simulink model "EXTENDEDKALMANFINAL2021abid"  (R2021a)
settings: Solver=ode4  StartTime=0.0  StopTime=200  FixedStep=0.02  RelTol=1e-3
libraries: commchan3 x2
(part 3 of 4)

== matlab function EXTENDEDKALMANFINAL2021abid/MATLAB Function2 ==
  data: xhatp input; Pp input; y input; u input; xhat output; P output
function [xhat, P]= fcn(xhatp, Pp, y, u)
x4=xhatp(4);
x5=xhatp(5);
x1=xhatp(1);
x2=xhatp(2);
x3=xhatp(3);

A=[                                                                                                                                                                                                                                                                                                                                                                             (x5/x4 + 5)/(1500000*x4) - 67/(505000*x4) + 1,                                                                                                                                                                                                                                                                                                                                                                                                                                                                                                                             ((x5/x4 + 5)*(x5/(20*x4) + 1/x4))/1500000 - x5/(150000*x4) - 1/(7500*x4) + 1/50,                                                                                                                                                                                                                                                                                                                                                                                                                                                                                                                                                  ((x5/x4 + 5)*(x5/(100*x4) - 19/20))/1500000 - (7*x5)/(10000000*x4) - 1/(1515000*x4) + 59/300000,                                                                                                                                                                                                                                                                                                                                                                                                                                                                                                                                                                                                                                                                                                                                                                                                                                                                                                                                                                                                                                                                                                                                                                                                                                                                                                                                                                                                                                                                                                                                                                                                                                                                                                                                                                                                                                                                                                                                                                                                                                                                                                                                                                                                                                                                                                                                                                                                                                                                                                                                                                                                                                                                                                                                                                                                                                                                                                                                                                                                                                                                                                                                                                                                                                       (x2*((5*x5)/x4^2 + 100/x4^2))/1500000 + (((5*x5)/x4^2 + 10000/(101*x4^2))*(x2 + x3/100))/1500000 - ((x5/x4 + 5)*((x2*((5*x5)/x4^2 + 100/x4^2))/100 + u/(20*x4^2) + x1/x4^2 + (x3*x5)/(100*x4^2)))/1500000 + (67*u)/(10100000*x4^2) + x1/(15000*x4^2) + (x1 + x2/100)/(15150*x4^2) + (x3*x5)/(1500000*x4^2) - (x5*((x2*((5*x5)/x4 + 100/x4))/100 - x3 + u/(20*x4) + x1/x4 + (x3*(x5/x4 + 5))/100))/(1500000*x4^2),                                                                                                                                                                                                                                                                                                                                                                                                                                                                                                                                                                                                                                                                                                                                                                                                                                                                                                                                                                                                                                                                                                                                                                                                                                                                                                                                                                                                                                                                                                                                                                                                                                                                                                                                                                                                                                                                                                                                                                                                                                                                                                                                                                            ((x5/x4 + 5)*(x2/(20*x4) + x3/(100*x4)))/1500000 - x2/(300000*x4) - x3/(1500000*x4) + ((x2*((5*x5)/x4 + 100/x4))/100 - x3 + u/(20*x4) + x1/x4 + (x3*(x5/x4 + 5))/100)/(1500000*x4) - (x2 + x3/100)/(300000*x4);
                                                                                                                                                                                                                                                               (x5/x4 + 5)/(15000*x4) - ((x5/x4 + 5)*((x5/x4 + 5)/(100*x4) - 100/(101*x4)))/15000 + ((5*x5)/x4 + 1000000/(10101*x4))/(1500000*x4) - 3040301/(153030150*x4),                                                                                                                                                                                                                                                                                                                                                                 ((x5/x4 + 5)*(x5/(20*x4) + 1/x4))/15000 + ((x5/x4 + 5)*(x5/(20*x4) - ((x5/x4 + 5)*(x5/(20*x4) + 1/x4))/100 + 1/x4))/15000 - x5/(1500*x4) - 10151/(757575*x4) + (((5*x5)/x4 + 1000000/(10101*x4))*(x5/(2000*x4) + 1/(100*x4) - 1))/15000 + 1,                                                                                                                                                                                                                                                                                                                                                                               ((x5/x4 + 5)*(x5/(100*x4) - 19/20))/15000 - ((x5/x4 + 5)*(((x5/x4 + 5)*(x5/(100*x4) - 19/20))/100 - x5/(2000*x4) - 1/(101*x4) + 1))/15000 - (7*x5)/(100000*x4) + ((x5/(10000*x4) - 19/2000)*((5*x5)/x4 + 1000000/(10101*x4)))/15000 - 5101/(76515075*x4) + 59/3000,                                                                                                                                                                                                                                                                                                                                                                                                                                                                                                                                                                                                                                                                                                                                                                                                                                                                                                                                                                                                                                                                                                                                                                                                                                                                                                                                                                                                                                                                                                                                                                                                                                                                                                                                                                                                                                                                                                                                                                                                                                                                                                                                                                                                                                                                                                                        (x2*((5*x5)/x4^2 + 100/x4^2))/15000 - (((5*x5)/x4^2 + 1000000/(10101*x4^2))*((x2*((5*x5)/x4 + 100/x4))/10000 - x3/100 - x2 + u/(2000*x4) + x1/(100*x4) + (x3*(x5/x4 + 5))/10000))/15000 + (((5*x5)/x4^2 + 10000/(101*x4^2))*(x2 + x3/100))/15000 - ((x5/x4 + 5)*((((5*x5)/x4^2 + 10000/(101*x4^2))*(x2 + x3/100))/100 - ((x5/x4 + 5)*((x2*((5*x5)/x4^2 + 100/x4^2))/100 + u/(20*x4^2) + x1/x4^2 + (x3*x5)/(100*x4^2)))/100 + (5*u)/(101*x4^2) + (100*(x1 + x2/100))/(101*x4^2) - (x5*((x2*((5*x5)/x4 + 100/x4))/100 - x3 + u/(20*x4) + x1/x4 + (x3*(x5/x4 + 5))/100))/(100*x4^2)))/15000 - ((x5/x4 + 5)*((x2*((5*x5)/x4^2 + 100/x4^2))/100 + u/(20*x4^2) + x1/x4^2 + (x3*x5)/(100*x4^2)))/15000 - (((5*x5)/x4 + 1000000/(10101*x4))*((x2*((5*x5)/x4^2 + 100/x4^2))/10000 + u/(2000*x4^2) + x1/(100*x4^2) + (x3*x5)/(10000*x4^2)))/15000 + (3040301*u)/(3060603000*x4^2) + x1/(150*x4^2) + (200*(x1 + x2/100 + x3/10000))/(30303*x4^2) + (2*(x1 + x2/100))/(303*x4^2) + (x3*x5)/(15000*x4^2) - (x5*((x2*((5*x5)/x4 + 100/x4))/100 - x3 + u/(20*x4) + x1/x4 + (x3*(x5/x4 + 5))/100))/(15000*x4^2) - (x5*((((5*x5)/x4 + 10000/(101*x4))*(x2 + x3/100))/100 - ((x5/x4 + 5)*((x2*((5*x5)/x4 + 100/x4))/100 - x3 + u/(20*x4) + x1/x4 + (x3*(x5/x4 + 5))/100))/100 - x3 + (5*u)/(101*x4) + (100*(x1 + x2/100))/(101*x4)))/(15000*x4^2),                                                                                                                                                                                                                                                                                                                                                                                                                                                                                                                                                                                                                                                                                                                                                                                                                                                                                                                                                                                                                                                                                                                                                                                                                                                                                                                                                                                                                                                                                                                                                                          ((x5/x4 + 5)*(x2/(20*x4) + x3/(100*x4)))/15000 + ((((5*x5)/x4 + 10000/(101*x4))*(x2 + x3/100))/100 - ((x5/x4 + 5)*((x2*((5*x5)/x4 + 100/x4))/100 - x3 + u/(20*x4) + x1/x4 + (x3*(x5/x4 + 5))/100))/100 - x3 + (5*u)/(101*x4) + (100*(x1 + x2/100))/(101*x4))/(15000*x4) + (((5*x5)/x4 + 1000000/(10101*x4))*(x2/(2000*x4) + x3/(10000*x4)))/15000 + ((x2*((5*x5)/x4 + 100/x4))/10000 - x3/100 - x2 + u/(2000*x4) + x1/(100*x4) + (x3*(x5/x4 + 5))/10000)/(3000*x4) - ((x5/x4 + 5)*(((x5/x4 + 5)*(x2/(20*x4) + x3/(100*x4)))/100 + ((x2*((5*x5)/x4 + 100/x4))/100 - x3 + u/(20*x4) + x1/x4 + (x3*(x5/x4 + 5))/100)/(100*x4) - (x2 + x3/100)/(20*x4)))/15000 - x2/(3000*x4) - x3/(15000*x4) + ((x2*((5*x5)/x4 + 100/x4))/100 - x3 + u/(20*x4) + x1/x4 + (x3*(x5/x4 + 5))/100)/(15000*x4) - (x2 + x3/100)/(3000*x4);
(x5/x4 + 5)/(150*x4) - ((x5/x4 + 5)*((x5/x4 + 5)/(100*x4) - 100/(101*x4)))/150 + ((5*x5)/x4 + 1000000/(10101*x4))/(15000*x4) - (((5*x5)/x4 + 50000000/(510101*x4))*((x5/x4 + 5)/(5000*x4) - 2/(101*x4)))/300 + ((x5/x4 + 5)*(((x5/x4 + 5)*((x5/x4 + 5)/(100*x4) - 100/(101*x4)))/50 - ((5*x5)/x4 + 1000000/(10101*x4))/(5000*x4) + 20000/(10101*x4)))/300 + (500000*(1/(5000*x4) - 1))/(1530303*x4) - 5060401/(3060603*x4), ((x5/x4 + 5)*(x5/(20*x4) + 1/x4))/150 - (((5*x5)/x4 + 50000000/(510101*x4))*(((x5/x4 + 5)*(x5/(20*x4) + 1/x4))/5000 - x5/(1000*x4) - 1/(50*x4) + 1))/300 + (500000*(x5/(100000*x4) + 1/(5000*x4) - 1/50))/(1530303*x4) - ((x5/x4 + 5)*(((x5/x4 + 5)*(x5/(20*x4) - ((x5/x4 + 5)*(x5/(20*x4) + 1/x4))/100 + 1/x4))/50 - 200/(10101*x4) + (((5*x5)/x4 + 1000000/(10101*x4))*(x5/(2000*x4) + 1/(100*x4) - 1))/50))/300 + ((x5/x4 + 5)*(x5/(20*x4) - ((x5/x4 + 5)*(x5/(20*x4) + 1/x4))/100 + 1/x4))/150 - x5/(20*x4) - 30503/(30303*x4) + (((5*x5)/x4 + 1000000/(10101*x4))*(x5/(2000*x4) + 1/(100*x4) - 1))/150, (500000*(x5/(500000*x4) - 19/100000))/(1530303*x4) - ((x5/x4 + 5)*(((x5/x4 + 5)*(x5/(100*x4) - 19/20))/100 - x5/(2000*x4) - 1/(101*x4) + 1))/150 - (((5*x5)/x4 + 50000000/(510101*x4))*(((x5/x4 + 5)*(x5/(100*x4) - 19/20))/5000 - x5/(100000*x4) - 1/(5050*x4) + 1/50))/300 + ((x5/x4 + 5)*(x5/(100*x4) - 19/20))/150 - (11*x5)/(3000*x4) + ((x5/(10000*x4) - 19/2000)*((5*x5)/x4 + 1000000/(10101*x4)))/150 - 20404/(3060603*x4) + ((x5/x4 + 5)*(((x5/x4 + 5)*(((x5/x4 + 5)*(x5/(100*x4) - 19/20))/100 - x5/(2000*x4) - 1/(101*x4) + 1))/50 - ((x5/(10000*x4) - 19/2000)*((5*x5)/x4 + 1000000/(10101*x4)))/50 + 2/(10101*x4) - 1))/300 + 59/60, ((x5/x4 + 5)*((((5*x5)/x4^2 + 1000000/(10101*x4^2))*((x2*((5*x5)/x4 + 100/x4))/10000 - x3/100 - x2 + u/(2000*x4) + x1/(100*x4) + (x3*(x5/x4 + 5))/10000))/50 + ((x5/x4 + 5)*((((5*x5)/x4^2 + 10000/(101*x4^2))*(x2 + x3/100))/100 - ((x5/x4 + 5)*((x2*((5*x5)/x4^2 + 100/x4^2))/100 + u/(20*x4^2) + x1/x4^2 + (x3*x5)/(100*x4^2)))/100 + (5*u)/(101*x4^2) + (100*(x1 + x2/100))/(101*x4^2) - (x5*((x2*((5*x5)/x4 + 100/x4))/100 - x3 + u/(20*x4) + x1/x4 + (x3*(x5/x4 + 5))/100))/(100*x4^2)))/50 + (((5*x5)/x4 + 1000000/(10101*x4))*((x2*((5*x5)/x4^2 + 100/x4^2))/10000 + u/(2000*x4^2) + x1/(100*x4^2) + (x3*x5)/(10000*x4^2)))/50 - (1000*u)/(10101*x4^2) - (20000*(x1 + x2/100 + x3/10000))/(10101*x4^2) + (x5*((((5*x5)/x4 + 10000/(101*x4))*(x2 + x3/100))/100 - ((x5/x4 + 5)*((x2*((5*x5)/x4 + 100/x4))/100 - x3 + u/(20*x4) + x1/x4 + (x3*(x5/x4 + 5))/100))/100 - x3 + (5*u)/(101*x4) + (100*(x1 + x2/100))/(101*x4)))/(50*x4^2)))/300 - (((5*x5)/x4^2 + 1000000/(10101*x4^2))*((x2*((5*x5)/x4 + 100/x4))/10000 - x3/100 - x2 + u/(2000*x4) + x1/(100*x4) + (x3*(x5/x4 + 5))/10000))/150 + (x2*((5*x5)/x4^2 + 100/x4^2))/300 - (500000*((x2*((5*x5)/x4^2 + 100/x4^2))/500000 + u/(100000*x4^2) + x1/(5000*x4^2) + (x3*x5)/(500000*x4^2)))/(1530303*x4) + (((5*x5)/x4^2 + 50000000/(510101*x4^2))*(x2 + x3/50 + ((x5/x4 + 5)*((x2*((5*x5)/x4 + 100/x4))/100 - x3 + u/(20*x4) + x1/x4 + (x3*(x5/x4 + 5))/100))/5000 - (((5*x5)/x4 + 10000/(101*x4))*(x2 + x3/100))/5000 - u/(1010*x4) - (2*(x1 + x2/100))/(101*x4)))/300 + (((5*x5)/x4^2 + 10000/(101*x4^2))*(x2 + x3/100))/150 - ((x5/x4 + 5)*((((5*x5)/x4^2 + 10000/(101*x4^2))*(x2 + x3/100))/100 - ((x5/x4 + 5)*((x2*((5*x5)/x4^2 + 100/x4^2))/100 + u/(20*x4^2) + x1/x4^2 + (x3*x5)/(100*x4^2)))/100 + (5*u)/(101*x4^2) + (100*(x1 + x2/100))/(101*x4^2) - (x5*((x2*((5*x5)/x4 + 100/x4))/100 - x3 + u/(20*x4) + x1/x4 + (x3*(x5/x4 + 5))/100))/(100*x4^2)))/150 - ((x5/x4 + 5)*((x2*((5*x5)/x4^2 + 100/x4^2))/100 + u/(20*x4^2) + x1/x4^2 + (x3*x5)/(100*x4^2)))/150 - (500000*((x2*((5*x5)/x4 + 100/x4))/500000 - x2/50 - x3/5000 - x1 + u/(100000*x4) + x1/(5000*x4) + (x3*(x5/x4 + 5))/500000))/(1530303*x4^2) - (((5*x5)/x4 + 50000000/(510101*x4))*((((5*x5)/x4^2 + 10000/(101*x4^2))*(x2 + x3/100))/5000 - ((x5/x4 + 5)*((x2*((5*x5)/x4^2 + 100/x4^2))/100 + u/(20*x4^2) + x1/x4^2 + (x3*x5)/(100*x4^2)))/5000 + u/(1010*x4^2) + (2*(x1 + x2/100))/(101*x4^2) - (x5*((x2*((5*x5)/x4 + 100/x4))/100 - x3 + u/(20*x4) + x1/x4 + (x3*(x5/x4 + 5))/100))/(5000*x4^2)))/300 - (((5*x5)/x4 + 1000000/(10101*x4))*((x2*((5*x5)/x4^2 + 100/x4^2))/10000 + u/(2000*x4^2) + x1/(100*x4^2) + (x3*x5)/(10000*x4^2)))/150 + (3091416110501*u)/(31224333018060*x4^2) + x1/(3*x4^2) + (20000*(x1 + x2/100 + x3/10000))/(30303*x4^2) + (200*(x1 + x2/100))/(303*x4^2) + (x3*x5)/(300*x4^2) - (x5*((x2*((5*x5)/x4 + 100/x4))/100 - x3 + u/(20*x4) + x1/x4 + (x3*(x5/x4 + 5))/100))/(150*x4^2) + (x5*(x3 + (((5*x5)/x4 + 1000000/(10101*x4))*((x2*((5*x5)/x4 + 100/x4))/10000 - x3/100 - x2 + u/(2000*x4) + x1/(100*x4) + (x3*(x5/x4 + 5))/10000))/50 + ((x5/x4 + 5)*((((5*x5)/x4 + 10000/(101*x4))*(x2 + x3/100))/100 - ((x5/x4 + 5)*((x2*((5*x5)/x4 + 100/x4))/100 - x3 + u/(20*x4) + x1/x4 + (x3*(x5/x4 + 5))/100))/100 - x3 + (5*u)/(101*x4) + (100*(x1 + x2/100))/(101*x4)))/50 - (1000*u)/(10101*x4) - (20000*(x1 + x2/100 + x3/10000))/(10101*x4)))/(300*x4^2) - (x5*((((5*x5)/x4 + 10000/(101*x4))*(x2 + x3/100))/100 - ((x5/x4 + 5)*((x2*((5*x5)/x4 + 100/x4))/100 - x3 + u/(20*x4) + x1/x4 + (x3*(x5/x4 + 5))/100))/100 - x3 + (5*u)/(101*x4) + (100*(x1 + x2/100))/(101*x4)))/(150*x4^2), ((x5/x4 + 5)*(x2/(20*x4) + x3/(100*x4)))/150 - (x3 + (((5*x5)/x4 + 1000000/(10101*x4))*((x2*((5*x5)/x4 + 100/x4))/10000 - x3/100 - x2 + u/(2000*x4) + x1/(100*x4) + (x3*(x5/x4 + 5))/10000))/50 + ((x5/x4 + 5)*((((5*x5)/x4 + 10000/(101*x4))*(x2 + x3/100))/100 - ((x5/x4 + 5)*((x2*((5*x5)/x4 + 100/x4))/100 - x3 + u/(20*x4) + x1/x4 + (x3*(x5/x4 + 5))/100))/100 - x3 + (5*u)/(101*x4) + (100*(x1 + x2/100))/(101*x4)))/50 - (1000*u)/(10101*x4) - (20000*(x1 + x2/100 + x3/10000))/(10101*x4))/(300*x4) + ((((5*x5)/x4 + 10000/(101*x4))*(x2 + x3/100))/100 - ((x5/x4 + 5)*((x2*((5*x5)/x4 + 100/x4))/100 - x3 + u/(20*x4) + x1/x4 + (x3*(x5/x4 + 5))/100))/100 - x3 + (5*u)/(101*x4) + (100*(x1 + x2/100))/(101*x4))/(150*x4) + (((5*x5)/x4 + 1000000/(10101*x4))*(x2/(2000*x4) + x3/(10000*x4)))/150 + ((x2*((5*x5)/x4 + 100/x4))/10000 - x3/100 - x2 + u/(2000*x4) + x1/(100*x4) + (x3*(x5/x4 + 5))/10000)/(30*x4) - ((x5/x4 + 5)*(((x5/x4 + 5)*(x2/(20*x4) + x3/(100*x4)))/100 + ((x2*((5*x5)/x4 + 100/x4))/100 - x3 + u/(20*x4) + x1/x4 + (x3*(x5/x4 + 5))/100)/(100*x4) - (x2 + x3/100)/(20*x4)))/150 - x2/(60*x4) - x3/(300*x4) + ((x2*((5*x5)/x4 + 100/x4))/100 - x3 + u/(20*x4) + x1/x4 + (x3*(x5/x4 + 5))/100)/(150*x4) - (x2 + x3/50 + ((x5/x4 + 5)*((x2*((5*x5)/x4 + 100/x4))/100 - x3 + u/(20*x4) + x1/x4 + (x3*(x5/x4 + 5))/100))/5000 - (((5*x5)/x4 + 10000/(101*x4))*(x2 + x3/100))/5000 - u/(1010*x4) - (2*(x1 + x2/100))/(101*x4))/(60*x4) - ((x5/x4 + 5)*(((((5*x5)/x4 + 10000/(101*x4))*(x2 + x3/100))/100 - ((x5/x4 + 5)*((x2*((5*x5)/x4 + 100/x4))/100 - x3 + u/(20*x4) + x1/x4 + (x3*(x5/x4 + 5))/100))/100 - x3 + (5*u)/(101*x4) + (100*(x1 + x2/100))/(101*x4))/(50*x4) + (((5*x5)/x4 + 1000000/(10101*x4))*(x2/(2000*x4) + x3/(10000*x4)))/50 + ((x2*((5*x5)/x4 + 100/x4))/10000 - x3/100 - x2 + u/(2000*x4) + x1/(100*x4) + (x3*(x5/x4 + 5))/10000)/(10*x4) - ((x5/x4 + 5)*(((x5/x4 + 5)*(x2/(20*x4) + x3/(100*x4)))/100 + ((x2*((5*x5)/x4 + 100/x4))/100 - x3 + u/(20*x4) + x1/x4 + (x3*(x5/x4 + 5))/100)/(100*x4) - (x2 + x3/100)/(20*x4)))/50))/300 - (((5*x5)/x4 + 50000000/(510101*x4))*(((x5/x4 + 5)*(x2/(20*x4) + x3/(100*x4)))/5000 + ((x2*((5*x5)/x4 + 100/x4))/100 - x3 + u/(20*x4) + x1/x4 + (x3*(x5/x4 + 5))/100)/(5000*x4) - (x2 + x3/100)/(1000*x4)))/300 - (x2 + x3/100)/(30*x4) + (500000*(x2/(100000*x4) + x3/(500000*x4)))/(1530303*x4);
                                                                                                                                                                                                                                                                                                                                                                                                                         0,                                                                                                                                                                                                                                                                                                                                                                                                                                                                                                                                                                                                           0,                                                                                                                                                                                                                                                                                                                                                                                                                                                                                                                                                                                                                                                0,                                                                                                                                                                                                                                                                                                                                                                                                                                                                                                                                                                                                                                                                                                                                                                                                                                                                                                                                                                                                                                                                                                                                                                                                                                                                                                                                                                                                                                                                                                                                                                                                                                                                                                                                                                                                                                                                                                                                                                                                                                                                                                                                                                                                                                                                                                                                                                                                                                                                                                                                                                                                                                                                                                                                                                                                                                                                                                                                                                                                                                                                                                                                                                                                                                                                                                                                                                                                                                                                                                                                                                                                                                      51010067/50000000,                                                                                                                                                                                                                                                                                                                                                                                                                                                                                                                                                                                                                                                                                                                                                                                                                                                                                                                                                                                                                                                                                                                                                                                                                                                                                                                                                                                                                                                                                                                                                                                                                                                                                                                                                                                                                                                                                                                                                                                                                                                                                                                                                                                                                                                                                                                                                                                         0;
                                                                                                                                                                                                                                                                                                                                                                                                                         0,                                                                                                                                                                                                                                                                                                                                                                                                                                                                                                                                                                                                           0,                                                                                                                                                                                                                                                                                                                                                                                                                                                                                                                                                                                                                                                0,                                                                                                                                                                                                                                                                                                                                                                                                                                                                                                                                                                                                                                                                                                                                                                                                                                                                                                                                                                                                                                                                                                                                                                                                                                                                                                                                                                                                                                                                                                                                                                                                                                                                                                                                                                                                                                                                                                                                                                                                                                                                                                                                                                                                                                                                                                                                                                                                                                                                                                                                                                                                                                                                                                                                                                                                                                                                                                                                                                                                                                                                                                                                                                                                                                                                                                                                                                                                                                                                                                                                                                                                                                                      0,                                                                                                                                                                                                                                                                                                                                                                                                                                                                                                                                                                                                                                                                                                                                                                                                                                                                                                                                                                                                                                                                                                                                                                                                                                                                                                                                                                                                                                                                                                                                                                                                                                                                                                                                                                                                                                                                                                                                                                                                                                                                                                                                                                                                                                                                                                                                                                         51010067/50000000];
 
B=[(x5/x4 + 5)/(30000000*x4) - 67/(10100000*x4);
                                                                                                                                                                                                                                                       (x5/x4 + 5)/(300000*x4) - ((x5/x4 + 5)*((x5/x4 + 5)/(2000*x4) - 5/(101*x4)))/15000 + ((5*x5)/x4 + 1000000/(10101*x4))/(30000000*x4) - 3040301/(3060603000*x4);
(x5/x4 + 5)/(3000*x4) - ((x5/x4 + 5)*((x5/x4 + 5)/(2000*x4) - 5/(101*x4)))/150 + ((5*x5)/x4 + 1000000/(10101*x4))/(300000*x4) - (((5*x5)/x4 + 50000000/(510101*x4))*((x5/x4 + 5)/(100000*x4) - 1/(1010*x4)))/300 + ((x5/x4 + 5)*(((x5/x4 + 5)*((x5/x4 + 5)/(2000*x4) - 5/(101*x4)))/50 - ((5*x5)/x4 + 1000000/(10101*x4))/(100000*x4) + 1000/(10101*x4)))/300 - 3091416110501/(31224333018060*x4) + 5/(1530303*x4^2);
                                                                                                                                                                                                                                                                                                                                                                                                                   0;
                                                                                                                                                                                                                                                                                                                                                                                                                   0];
% Pa = reshape(Pp,[3,3]);

Pa = reshape(Pp, [5, 5]);

Q=eye(5,5)*1e-7;
R=1e-6;
C=[0, 1, 0,0,0];
%Prior State  
xhatprior= Fd1(xhatp,y,0.02);  %
Pkprior= A*Pa*A' + Q;

%Posterior State
K=(Pkprior*C')/(C*Pkprior*C'+R);
xhat=xhatprior+K*(y-C*xhatprior);
P=reshape((eye(5)-K*C)*Pkprior, [25,1]);



function dotX1 = Fc1(x, u)
    x1 = x(1); 
    x2 = x(2);
    x3 =x(3);
    M = x(4);
    D = x(5);
    Tg = 0.2;
    Rp = 0.05;
    Ki=2;
    %C = Param(3);
    u = u(1);
    dotX1 = [x2;x3;-Ki*M/(Tg)*x1-(D*M/(Tg)+M/(Rp*Tg))*x2-(D*M+1/Tg)*x3-M/(Tg)*u;0;0];
       
end
% Discretized equations
function x_1 = Fd1(x, u,Ts)
    k1 = Fc1(x, u);
    k2 = Fc1(x + Ts/2*k1, u);
    k3 = Fc1(x + Ts/2*k2, u);
    k4 = Fc1(x + Ts*k3, u);
    x_1 = x + Ts/6*(k1 + 2*k2 + 2*k3+k4);
end
end
